simulink subsystem "VehicleSimulationRef"  (R2024a)
settings: Solver=VariableStepAuto  StartTime=0.0  StopTime=10.0  RelTol=1e-3
undefined symbols (not defined in the file): damp, Ka_accel, Kd_rate, Ki_angle, Kp_angle, omega, SimIn, SimPar
libraries: simulink_extras x3, vrlib x3, aerolibanimutils x1, simulink x1
settings Model: Creator=tbritton  LastModifiedBy=adcl
settings SolverCC: AlgebraicLoopSolver=TrustRegion
settings OptimizationCC: ReuseModelBlockBuffer=off
settings DebuggingCC: UnconnectedInputMsg=warning  UnconnectedOutputMsg=warning  UnconnectedLineMsg=warning
settings ModelReferenceCC: EnableRefExpFcnMdlSchedulingChecks=on
settings RTWCC: GPUComputeCapability=3.5  DLArmComputeVersion=19.05

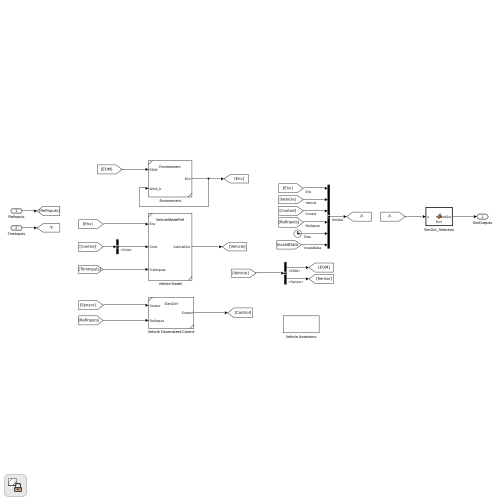
[thumbnail: Simulink's stored preview of the top-level diagram]
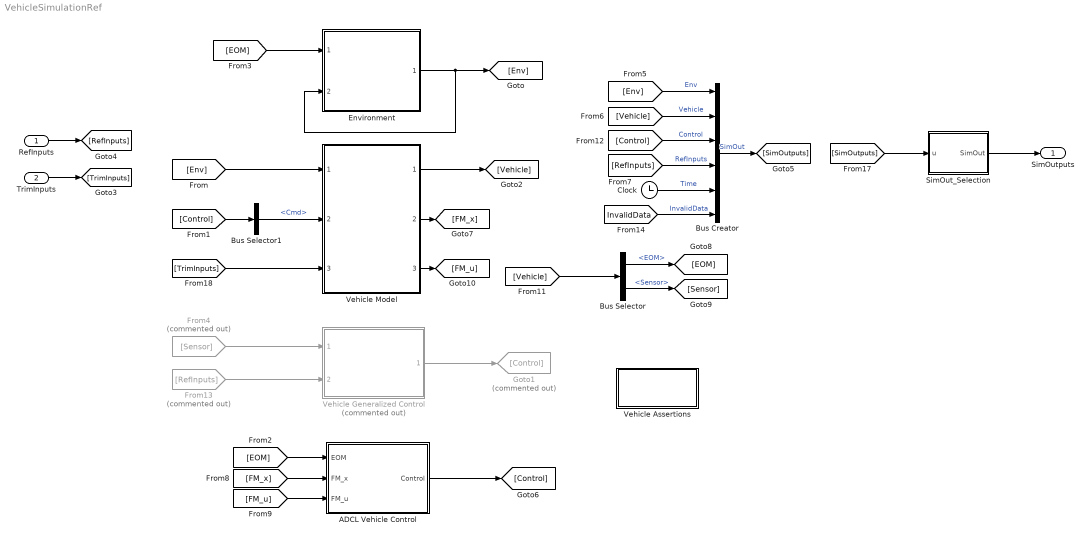
== system VehicleSimulationRef ==
  RefInputs : Inport  OutDataTypeStr=Bus: BUS_REF_INPUT
  TrimInputs : Inport  Port=2  OutDataTypeStr=Bus: BUS_TRIM_INPUT
  ADCL Vehicle Control : Subsystem
  Bus Creator : BusCreator  Inputs=6  OutDataTypeStr=Bus: BUS_SIM_OUT  NonVirtualBus=on
  Bus Selector : BusSelector  OutputSignals=EOM,Sensor
  Bus Selector1 : BusSelector  OutputSignals=Cmd
  Clock : Clock
  Environment : Subsystem  ReferencedSubsystem=Environment
  From13 : From  Commented=on  GotoTag=RefInputs
  From4 : From  Commented=on  GotoTag=Sensor
  Goto1 : Goto  Commented=on  GotoTag=Control
  SimOut_Selection : MATLAB Function  TreatAsAtomicUnit=on
  Vehicle Assertions : Subsystem
  Vehicle Generalized Control : Subsystem  Commented=on  ReferencedSubsystem=GenCtrl
  Vehicle Model : Subsystem  ReferencedSubsystem=VehicleModelRef
  SimOutputs : Outport  OutDataTypeStr=Bus: BUS_USER_SIM_OUT
  wires:
  From4/1 -> Vehicle Generalized Control/1
  [Env] -> Bus Creator/1  "Env"
  [RefInputs] -> Bus Creator/4  "RefInputs"
  Environment/1 -> [Env], Environment/2
  Vehicle Generalized Control/1 -> Goto1/1
  [Vehicle] -> Bus Creator/2  "Vehicle"
  [Control] -> Bus Creator/3  "Control"
  Bus Selector/1 -> [EOM]  "<EOM>"
  [Vehicle] -> Bus Selector/1
  [EOM] -> Environment/1
  Bus Selector/2 -> [Sensor]  "<Sensor>"
  [Control] -> Bus Selector1/1
  From13/1 -> Vehicle Generalized Control/2
  Clock/1 -> Bus Creator/5  "Time"
  TrimInputs/1 -> [TrimInputs]
  RefInputs/1 -> [RefInputs]
  Bus Creator/1 -> [SimOutputs]  "SimOut"
  [InvalidData] -> Bus Creator/6  "InvalidData"
  [Env] -> Vehicle Model/1
  Bus Selector1/1 -> Vehicle Model/2  "<Cmd>"
  [TrimInputs] -> Vehicle Model/3
  Vehicle Model/1 -> [Vehicle]
  [SimOutputs] -> SimOut_Selection/1(u)
  SimOut_Selection/1(SimOut) -> SimOutputs/1
  [EOM] -> ADCL Vehicle Control/1(EOM)
  ADCL Vehicle Control/1(Control) -> [Control]
  [FM_x] -> ADCL Vehicle Control/2(FM_x)
  [FM_u] -> ADCL Vehicle Control/3(FM_u)
  Vehicle Model/3 -> [FM_u]
  Vehicle Model/2 -> [FM_x]

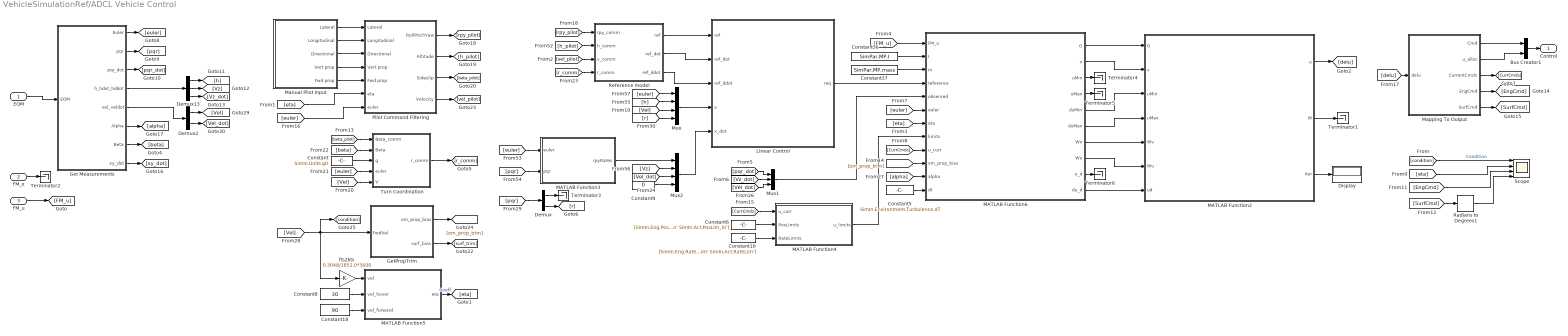
== system VehicleSimulationRef/ADCL Vehicle Control ==
  EOM : Inport
  FM_x : Inport  Port=2
  FM_u : Inport  Port=3
  Bus Creator1 : BusCreator  Inputs=2
  Constant : Constant  Value=SimIn.Units.g0
  Constant10 : Constant  Value=[SimIn.Eng.RateLim' SimIn.Act.RateLim']
  Constant18 : Constant  Value=90
  Constant36 : Constant  Value=SimPar.MP.I
  Constant37 : Constant  Value=SimPar.MP.mass
  Constant5 : Constant  Value=SimIn.Environment.Turbulence.dT
  Constant6 : Constant  Value=[SimIn.Eng.PosLim_hi' SimIn.Act.PosLim_hi'; SimIn.Eng.PosLim_lo' SimIn.Act.PosLim_lo']
  Constant8 : Constant  Value=30
  Constant9 : Constant  Value=0
  Demux : Demux  Outputs=[2 1]
  Demux13 : Demux  Outputs=3
  Demux2 : Demux  Outputs=2
  Display : Display
  Get Measurements : Subsystem
  GetPropTrim : Subsystem
  Linear Control : Subsystem  mask{Krp_angle=5, Krp_angle_i=3, Krp_rate=5, Krp_accel=1, Ky_angle=0.75, Ky_rate=2.5, Ky_accel=0.75, Kr_rate=2, Kh_angle=0.8, Kh_rate=2, Kh_accel=1}
      mask prompts: Krp_angle "Roll and Pitch angle gain"; Krp_angle_i "Roll and Pitch angle gain integral"; Krp_rate "Roll and Pitch rate gain"; Krp_accel "Roll and Pitch accel. gain"; Ky_angle "Yaw angle gain"; Ky_rate "Yaw rate gain"; Ky_accel "Yaw accel. gain"; Kr_rate "Turn coord. rate gain"; Kh_angle "Altitude angle gain"; Kh_rate "Altitude rate gain"; Kh_accel "Altitude accel. gain"
      mask DialogControl DescTextVar Prompt: Linear controller gains
      mask DialogControl Container3 Prompt: Roll and Pitch
      mask DialogControl Container4 Prompt: Yaw
      mask DialogControl Container5 Prompt: Altitude and Forward vel.
  MATLAB Function2 : MATLAB Function  TreatAsAtomicUnit=on
  MATLAB Function3 : MATLAB Function  TreatAsAtomicUnit=on
  MATLAB Function4 : MATLAB Function  TreatAsAtomicUnit=on
  MATLAB Function5 : MATLAB Function  TreatAsAtomicUnit=on
  MATLAB Function6 : MATLAB Function  TreatAsAtomicUnit=on
  Manual Pilot Input : Subsystem
  Mapping To Output : Subsystem
  Mux : Mux
  Mux1 : Mux  Inputs=3
  Mux2 : Mux
  Pilot Command Filtering : Subsystem
  Radians to Degrees1 : simulink_extras/Transformations/Radians to Degrees
  Reference model : Subsystem  mask{r_omega=1.4, r_damp=0.8, p_omega=2.4, p_damp=0.8, y_omega=0.67, y_damp=0.8, h_omega=0.67, h_damp=0.8}
      mask prompts: r_omega "Roll natural freq."; r_damp "Roll damping ratio"; p_omega "Pitch natural freq."; p_damp "Pitch damping ratio"; y_omega "Yaw natural freq."; y_damp "Yaw damping ratio"; h_omega "Altitude natural freq."; h_damp "Altitude damping ratio"
      mask DialogControl DescTextVar Prompt: Second order reference models for the roll, pitch, yaw and altitude channles
      mask DialogControl Container3 Prompt: Roll parameters
      mask DialogControl Container4 Prompt: Pitch parameters
      mask DialogControl Container5 Prompt: Yaw parameters
      mask DialogControl Container6 Prompt: Altitude parameters
  Scope : Scope  NumInputPorts=4
  Terminator{1..6} (6 alike) : Terminator
  Turn Coordination : Subsystem  mask{Kbeta=0.5}
      mask prompts: Kbeta "Controller gain"
      mask DialogControl DescTextVar Prompt: Sideslip control for turn coordination
  fts2kts : Gain  Gain=0.3048/1852.0*3600
  Control : Outport
  wires:
  MATLAB Function6/3(uMin) -> Terminator4/1
  MATLAB Function6/4(uMax) -> Terminator5/1
  MATLAB Function6/9(u_d) -> Terminator6/1
  Pilot Command Filtering/1(RollPitchYaw) -> [rpy_pilot]
  Pilot Command Filtering/2(Altitude) -> [h_pilot]
  Pilot Command Filtering/3(Sideslip) -> [beta_pilot]
  Pilot Command Filtering/4(Velocity) -> [vel_pilot]
  [euler] -> Pilot Command Filtering/7(euler)
  [eta] -> Pilot Command Filtering/6(eta)
  Manual Pilot Input/5(Fwd prop) -> Pilot Command Filtering/5(Fwd prop)
  Manual Pilot Input/4(Vert prop) -> Pilot Command Filtering/4(Vert prop)
  Manual Pilot Input/3(Directional) -> Pilot Command Filtering/3(Directional)
  Manual Pilot Input/2(Longitudinal) -> Pilot Command Filtering/2(Longitudinal)
  Manual Pilot Input/1(Lateral) -> Pilot Command Filtering/1(Lateral)
  [h] -> Mux/2
  EOM/1 -> Get Measurements/1(EOM)
  Mux/1 -> Linear Control/4(x)
  [h_pilot] -> Reference model/2(h_comm)
  Reference model/2(ref_dot) -> Linear Control/2(ref_dot)
  Reference model/3(ref_ddot) -> Linear Control/3(ref_ddot)
  [euler] -> MATLAB Function3/1(euler)
  Mux2/1 -> Linear Control/5(x_dot)
  Reference model/1(ref) -> Linear Control/1(ref)
  [pqr] -> MATLAB Function3/2(pqr)
  [euler] -> Mux/1
  [Vz] -> Mux2/2
  [rpy_pilot] -> Reference model/1(rpy_comm)
  MATLAB Function3/1(rpyRates) -> Mux2/1
  Bus Creator1/1 -> Control/1
  FM_x/1 -> Terminator2/1
  FM_u/1 -> [FM_u]
  [FM_u] -> MATLAB Function6/1(FM_u)
  Constant36/1 -> MATLAB Function6/2(I)
  Constant37/1 -> MATLAB Function6/3(m)
  [eta] -> MATLAB Function6/7(eta)
  [euler] -> MATLAB Function6/6(euler)
  MATLAB Function6/2(v) -> MATLAB Function2/2(v)
  [eta] -> Scope/2
  [SurfCmd] -> Radians to Degrees1/1
  [EngCmd] -> Scope/3
  Radians to Degrees1/1 -> Scope/4
  Get Measurements/4(h_hdot_hddot) -> Demux13/1
  Get Measurements/1(Euler) -> [euler]
  Get Measurements/2(pqr) -> [pqr]
  Get Measurements/3(pqr_dot) -> [pqr_dot]
  Demux13/1 -> [h]
  Demux13/2 -> [Vz]
  Demux13/3 -> [Vz_dot]
  Get Measurements/6(Alpha) -> [alpha]
  [om_prop_trim] -> MATLAB Function6/10(om_prop_bias)
  Mapping To Output/1(Cmd) -> Bus Creator1/1
  Mapping To Output/2(u_alloc) -> Bus Creator1/2
  Mapping To Output/3(CurrentCmds) -> [CurrCmds]
  [CurrCmds] -> MATLAB Function6/9(u_curr)
  Mapping To Output/5(SurfCmd) -> [SurfCmd]
  Mapping To Output/4(EngCmd) -> [EngCmd]
  Linear Control/1(req) -> MATLAB Function6/4(reference)
  Get Measurements/5(vel_veldot) -> Demux2/1
  Demux2/2 -> [Vel_dot]
  Demux2/1 -> [Vel]
  [Vel] -> Mux/3
  [Vel_dot] -> Mux2/3
  [alpha] -> MATLAB Function6/11(alpha)
  MATLAB Function6/1(G) -> MATLAB Function2/1(G)
  MATLAB Function6/7(Wv) -> MATLAB Function2/5(Wv)
  MATLAB Function6/8(Wu) -> MATLAB Function2/6(Wu)
  MATLAB Function6/5(duMin) -> MATLAB Function2/3(uMin)
  MATLAB Function6/6(duMax) -> MATLAB Function2/4(uMax)
  MATLAB Function5/1(eta) -> [eta]  "Coeff"
  [Vz_dot] -> Mux1/2
  [pqr_dot] -> Mux1/1
  [Vel_dot] -> Mux1/3
  Constant5/1 -> MATLAB Function6/12(dt)
  [vel_pilot] -> Reference model/3(v_comm)
  Constant6/1 -> MATLAB Function4/2(PosLimits)
  MATLAB Function4/1(u_limits) -> MATLAB Function6/8(limits)
  GetPropTrim/1(om_prop_bias) -> [om_prop_trim]
  MATLAB Function6/10(du_d) -> MATLAB Function2/7(ud)
  [Vel] -> GetPropTrim/1(FwdVel), [condition], fts2kts/1
  fts2kts/1 -> MATLAB Function5/1(vel)
  Constant8/1 -> MATLAB Function5/2(vel_hover)
  Constant18/1 -> MATLAB Function5/3(vel_forward)
  GetPropTrim/2(surf_bias) -> [surf_trim]
  [condition] -> Scope/1  "Condition"
  MATLAB Function2/3(iter) -> Display/1
  MATLAB Function2/2(W) -> Terminator1/1
  [delu] -> Mapping To Output/1(delu)
  [CurrCmds] -> MATLAB Function4/1(u_curr)
  Mux1/1 -> MATLAB Function6/5(observed)
  MATLAB Function2/1(u) -> [delu]
  Constant10/1 -> MATLAB Function4/3(RateLimits)
  [beta_pilot] -> Turn Coordination/1(Beta_comm)
  [Vel] -> Turn Coordination/5(V)
  [euler] -> Turn Coordination/4(euler)
  Get Measurements/7(Beta) -> [beta]
  [beta] -> Turn Coordination/2(Beta)
  Constant/1 -> Turn Coordination/3(g)
  [r_comm] -> Reference model/4(r_comm)
  [pqr] -> Demux/1
  Demux/2 -> [r]
  Demux/1 -> Terminator3/1
  [r] -> Mux/4
  Constant9/1 -> Mux2/4
  Turn Coordination/1(r_comm) -> [r_comm]
  Get Measurements/8(xy_dot) -> [xy_dot]

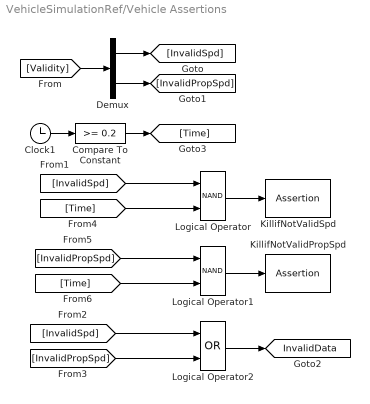
== system VehicleSimulationRef/Vehicle Assertions ==
  Clock1 : Clock
  Compare To Constant : simulink/Logic and Bit Operations/Compare To Constant  relop=>=  const=0.2  OutDataTypeStr=boolean  ZeroCross=off
  Demux : Demux  Outputs=2
  KillifNotValidPropSpd : Assertion  AssertionFailFcn=warndlg('Model invalid prop speeds','Warning!')
  KillifNotValidSpd : Assertion  AssertionFailFcn=warndlg('Model invalid speed','Warning!')
  Logical Operator : Logic  Operator=NAND  AllPortsSameDT=off  OutDataTypeStr=boolean
  Logical Operator1 : Logic  Operator=NAND  AllPortsSameDT=off  OutDataTypeStr=boolean
  Logical Operator2 : Logic  Operator=OR  AllPortsSameDT=off  OutDataTypeStr=boolean
  tag scope: InvalidData=global
  wires:
  [InvalidPropSpd] -> Logical Operator2/2
  [InvalidSpd] -> Logical Operator2/1
  Logical Operator2/1 -> [InvalidData]
  Logical Operator/1 -> KillifNotValidSpd/1
  [InvalidPropSpd] -> Logical Operator1/1
  Logical Operator1/1 -> KillifNotValidPropSpd/1
  [Time] -> Logical Operator1/2
  [Time] -> Logical Operator/2
  Compare To Constant/1 -> [Time]
  Demux/2 -> [InvalidPropSpd]
  Demux/1 -> [InvalidSpd]
  [Validity] -> Demux/1
  [InvalidSpd] -> Logical Operator/1
  Clock1/1 -> Compare To Constant/1

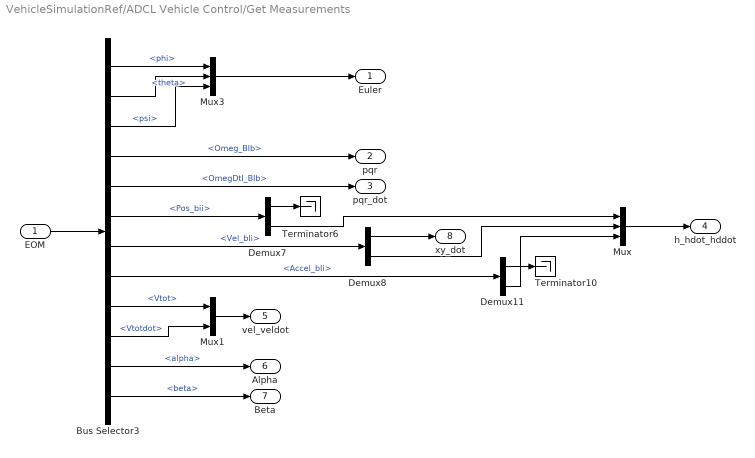
== system VehicleSimulationRef/ADCL Vehicle Control/Get Measurements ==
  EOM : Inport
  Bus Selector3 : BusSelector  OutputSignals=WorldRelativeData.Euler.phi,WorldRelativeData.Euler.theta,WorldRelativeData.Euler.psi,InertialData.Omeg_BIb,InertialData.OmegDtI_BIb,InertialData.Pos_bii,InertialData.Vel_bIi,InertialData.Accel_bIi,AirRelativeData.Vtot,AirRelativeData.Vtotdot,AirRelativeData.alpha,AirRelativeData.beta
  Demux11 : Demux  Outputs=[2 1]
  Demux7 : Demux  Outputs=[2 1]
  Demux8 : Demux  Outputs=[2 1]
  Mux : Mux  Inputs=3
  Mux1 : Mux  Inputs=2
  Mux3 : Mux  Inputs=3
  Terminator10 : Terminator
  Terminator6 : Terminator
  Euler : Outport
  pqr : Outport  Port=2
  pqr_dot : Outport  Port=3
  h_hdot_hddot : Outport  Port=4
  vel_veldot : Outport  Port=5
  Alpha : Outport  Port=6
  Beta : Outport  Port=7
  xy_dot : Outport  Port=8
  wires:
  Bus Selector3/7 -> Demux8/1  "<Vel_bIi>"
  Bus Selector3/6 -> Demux7/1  "<Pos_bii>"
  EOM/1 -> Bus Selector3/1
  Demux7/1 -> Terminator6/1
  Bus Selector3/8 -> Demux11/1  "<Accel_bIi>"
  Bus Selector3/1 -> Mux3/1  "<phi>"
  Demux11/1 -> Terminator10/1
  Demux11/2 -> Mux/3
  Demux7/2 -> Mux/1
  Bus Selector3/2 -> Mux3/2  "<theta>"
  Bus Selector3/3 -> Mux3/3  "<psi>"
  Mux3/1 -> Euler/1
  Bus Selector3/4 -> pqr/1  "<Omeg_BIb>"
  Bus Selector3/5 -> pqr_dot/1  "<OmegDtI_BIb>"
  Mux/1 -> h_hdot_hddot/1
  Demux8/2 -> Mux/2
  Bus Selector3/11 -> Alpha/1  "<alpha>"
  Bus Selector3/10 -> Mux1/2  "<Vtotdot>"
  Bus Selector3/9 -> Mux1/1  "<Vtot>"
  Mux1/1 -> vel_veldot/1
  Bus Selector3/12 -> Beta/1  "<beta>"
  Demux8/1 -> xy_dot/1

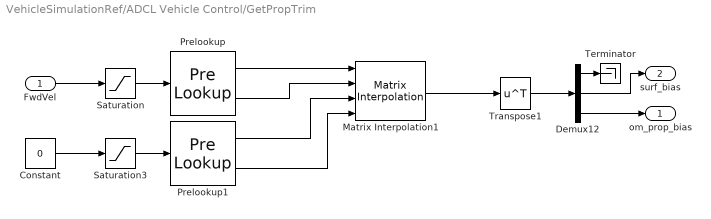
== system VehicleSimulationRef/ADCL Vehicle Control/GetPropTrim ==
  FwdVel : Inport
  Constant : Constant  Value=0
  Demux12 : Demux  Outputs=[12 4 9]
  Matrix Interpolation1 : simulink_extras/Additional Lookup Tables/Matrix Interpolation  InterpMethod=Linear  ExtrapMethod=Clip  InterpolateDimension=2  TableData=SimIn.Control.trim.XU0_interp  SimulateUsing=Code generation
  Prelookup : PreLookup  BreakpointsData=SimIn.Control.trim.UH
  Prelookup1 : PreLookup  BreakpointsData=SimIn.Control.trim.WH
  Saturation : Saturate  UpperLimit=178  LowerLimit=0
  Saturation3 : Saturate  UpperLimit=8.33  LowerLimit=-8.33
  Terminator : Terminator
  Transpose1 : Math  Operator=transpose
  om_prop_bias : Outport
  surf_bias : Outport  Port=2
  wires:
  Constant/1 -> Saturation3/1
  Prelookup/1 -> Matrix Interpolation1/1
  Prelookup1/1 -> Matrix Interpolation1/3
  Demux12/2 -> surf_bias/1
  Demux12/3 -> om_prop_bias/1
  Demux12/1 -> Terminator/1
  Prelookup/2 -> Matrix Interpolation1/2
  Prelookup1/2 -> Matrix Interpolation1/4
  Transpose1/1 -> Demux12/1
  Saturation/1 -> Prelookup/1
  Saturation3/1 -> Prelookup1/1
  FwdVel/1 -> Saturation/1
  Matrix Interpolation1/1 -> Transpose1/1

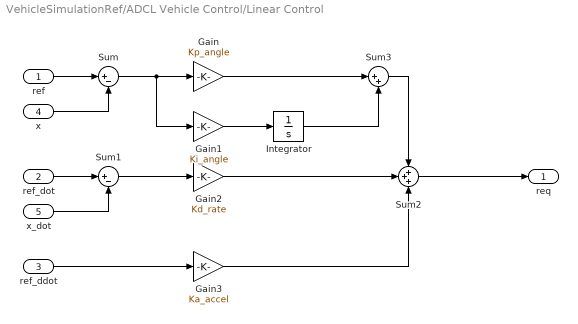
== system VehicleSimulationRef/ADCL Vehicle Control/Linear Control ==
  ref : Inport
  ref_dot : Inport  Port=2
  ref_ddot : Inport  Port=3
  x : Inport  Port=4
  x_dot : Inport  Port=5
  Gain : Gain  Gain=Kp_angle
  Gain1 : Gain  Gain=Ki_angle
  Gain2 : Gain  Gain=Kd_rate
  Gain3 : Gain  Gain=Ka_accel
  Integrator : Integrator
  Sum : Sum  Inputs=|+-
  Sum1 : Sum  Inputs=|+-
  Sum2 : Sum  Inputs=+++
  Sum3 : Sum  Inputs=|++
  req : Outport
  wires:
  ref/1 -> Sum/1
  x/1 -> Sum/2
  Gain1/1 -> Integrator/1
  Sum/1 -> Gain/1, Gain1/1
  ref_dot/1 -> Sum1/1
  Sum1/1 -> Gain2/1
  x_dot/1 -> Sum1/2
  ref_ddot/1 -> Gain3/1
  Gain3/1 -> Sum2/3
  Gain2/1 -> Sum2/2
  Gain/1 -> Sum3/1
  Integrator/1 -> Sum3/2
  Sum3/1 -> Sum2/1
  Sum2/1 -> req/1

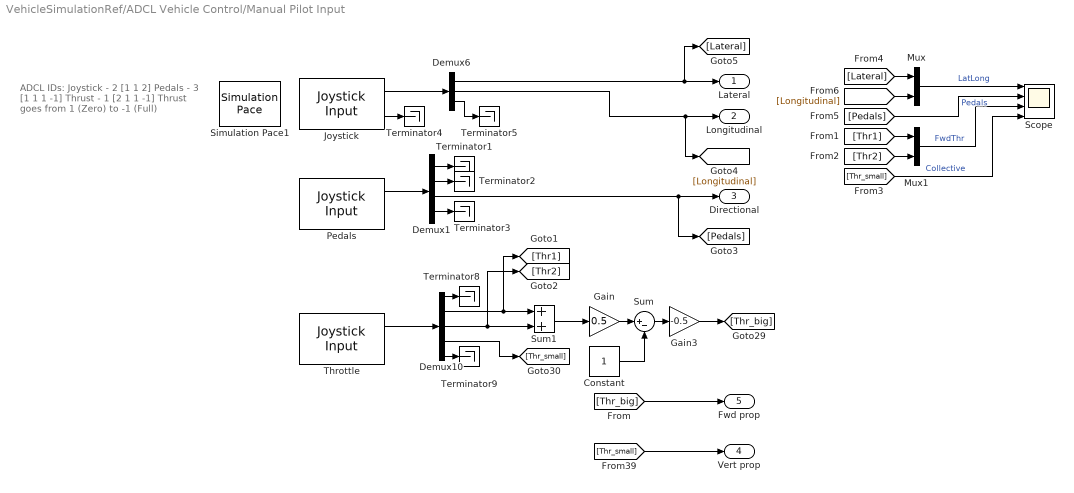
== system VehicleSimulationRef/ADCL Vehicle Control/Manual Pilot Input ==
  note: ADCL IDs:
      | Joystick - 2 [1 1 2]
      | Pedals - 3 [1 1 1 -1]
      | Thrust - 1 [2 1 1 -1]
      |
      | Thrust goes from 1 (Zero) to -1 (Full)
  Constant : Constant
  Demux1 : Demux  Outputs=[1 1 1 -1]
  Demux10 : Demux  Outputs=[2 1 1 1 2]
  Demux6 : Demux  Outputs=[1 1 2]
  Gain : Gain  Gain=0.5
  Gain3 : Gain  Gain=-0.5
  Joystick : vrlib/Joystick Input  joyid=2  adjustports=on  forcefeed=off
  Mux : Mux  Inputs=2
  Mux1 : Mux  Inputs=2
  Pedals : vrlib/Joystick Input  joyid=3  adjustports=off  forcefeed=off
  Scope : Scope  NumInputPorts=4
  Simulation Pace1 : aerolibanimutils/Simulation Pace  SimulationPace=1  SleepMode=Auto  OutputPaceError=off  SampleTime=SimIn.Environment.Turbulence.dT
  Sum : Sum  Inputs=|+-
  Sum1 : Sum
  Terminator{1..5,8..9} (7 alike) : Terminator
  Throttle : vrlib/Joystick Input  joyid=1  adjustports=on  forcefeed=off
  Lateral : Outport
  Longitudinal : Outport  Port=2
  Directional : Outport  Port=3
  Vert prop : Outport  Port=4
  Fwd prop : Outport  Port=5
  wires:
  [Thr_small] -> Scope/4  "Collective"
  Mux1/1 -> Scope/3  "FwdThr"
  [Pedals] -> Scope/2  "Pedals"
  Mux/1 -> Scope/1  "LatLong"
  [Thr2] -> Mux1/2
  [Thr1] -> Mux1/1
  [Lateral] -> Mux/1
  [Longitudinal] -> Mux/2
  Demux1/3 -> Directional/1, [Pedals]
  [Thr_small] -> Vert prop/1
  [Thr_big] -> Fwd prop/1
  Demux6/2 -> Longitudinal/1, [Longitudinal]
  Demux1/1 -> Terminator1/1
  Demux1/2 -> Terminator2/1
  Demux1/4 -> Terminator3/1
  Pedals/1 -> Demux1/1
  Gain3/1 -> [Thr_big]
  Constant/1 -> Sum/2
  Sum/1 -> Gain3/1
  Demux6/3 -> Terminator5/1
  Demux6/1 -> Lateral/1, [Lateral]
  Joystick/1 -> Demux6/1
  Throttle/1 -> Demux10/1
  Sum1/1 -> Gain/1
  Demux10/2 -> Sum1/1, [Thr1]
  Demux10/5 -> Terminator9/1
  Gain/1 -> Sum/1
  Demux10/1 -> Terminator8/1
  Demux10/3 -> Sum1/2, [Thr2]
  Demux10/4 -> [Thr_small]
  Joystick/2 -> Terminator4/1

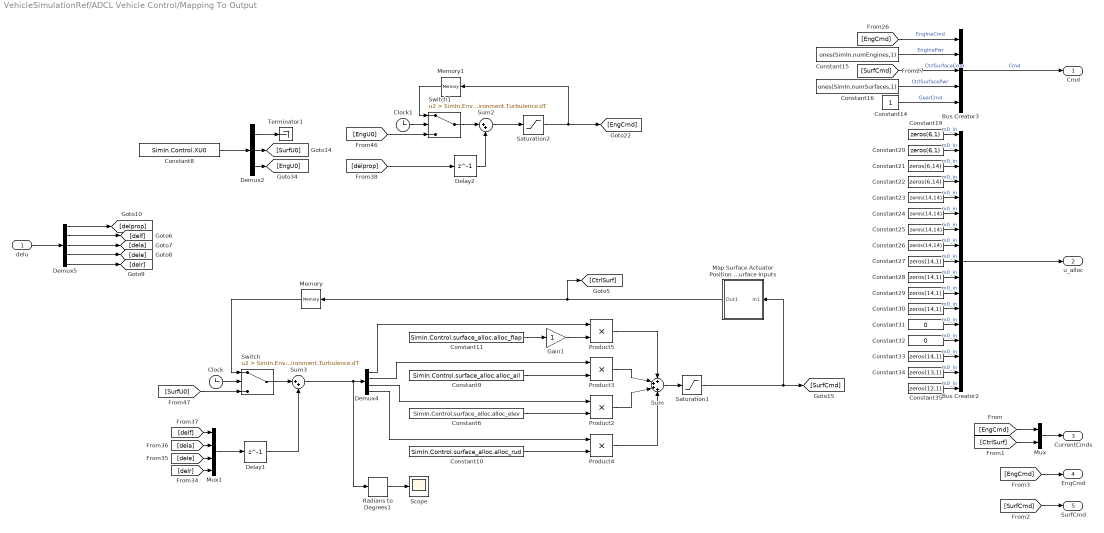
== system VehicleSimulationRef/ADCL Vehicle Control/Mapping To Output ==
  delu : Inport
  Bus Creator2 : BusCreator  Inputs=17  OutDataTypeStr=Bus: BUS_ALLOC
  Bus Creator3 : BusCreator  Inputs=5  OutDataTypeStr=Bus: BUS_CMD
  Clock : Clock
  Clock1 : Clock
  Constant10 : Constant  Value=SimIn.Control.surface_alloc.alloc_rud
  Constant11 : Constant  Value=SimIn.Control.surface_alloc.alloc_flap
  Constant14 : Constant
  Constant15 : Constant  Value=ones(SimIn.numEngines,1)
  Constant16 : Constant  Value=ones(SimIn.numSurfaces,1)
  Constant19 : Constant  Value=zeros(6,1)
  Constant20 : Constant  Value=zeros(6,1)
  Constant21 : Constant  Value=zeros(6,14)
  Constant22 : Constant  Value=zeros(6,14)
  Constant{23..26} (4 alike) : Constant  Value=zeros(14,14)
  Constant{27..30,33} (5 alike) : Constant  Value=zeros(14,1)
  Constant31 : Constant  Value=0
  Constant32 : Constant  Value=0
  Constant34 : Constant  Value=zeros(13,1)
  Constant35 : Constant  Value=zeros(12,1)
  Constant6 : Constant  Value=SimIn.Control.surface_alloc.alloc_elev
  Constant8 : Constant  Value=SimIn.Control.XU0
  Constant9 : Constant  Value=SimIn.Control.surface_alloc.alloc_ail
  Delay1 : Delay  DelayLength=1
  Delay2 : Delay  DelayLength=1
  Demux2 : Demux  Outputs=[-1 4 9]
  Demux4 : Demux
  Demux5 : Demux  Outputs=[9 1 1 1 1]
  Gain1 : Gain
  Map Surface Actuator Position To Surface Inputs : Subsystem
  Memory : Memory
  Memory1 : Memory
  Mux : Mux  Inputs=2
  Mux1 : Mux
  Product{2..5} (4 alike) : Product
  Radians to Degrees1 : simulink_extras/Transformations/Radians to Degrees
  Saturation1 : Saturate  UpperLimit=SimPar.Actuator.MaxPos  LowerLimit=SimPar.Actuator.MinPos
  Saturation2 : Saturate  UpperLimit=SimPar.Engine.MaxPos  LowerLimit=SimPar.Engine.MinPos
  Scope : Scope
  Sum : Sum  Inputs=++++
  Sum2 : Sum  Inputs=|++
  Sum3 : Sum  Inputs=|++
  Switch : Switch  Criteria=u2 > Threshold  Threshold=SimIn.Environment.Turbulence.dT  SaturateOnIntegerOverflow=off  InputSameDT=off
  Switch1 : Switch  Criteria=u2 > Threshold  Threshold=SimIn.Environment.Turbulence.dT  SaturateOnIntegerOverflow=off  InputSameDT=off
  Terminator1 : Terminator
  Cmd : Outport
  u_alloc : Outport  Port=2
  CurrentCmds : Outport  Port=3
  EngCmd : Outport  Port=4
  SurfCmd : Outport  Port=5
  wires:
  Constant6/1 -> Product2/2
  Switch/1 -> Sum3/1
  Bus Creator3/1 -> Cmd/1  "Cmd"
  Demux4/2 -> Product3/1
  Constant31/1 -> Bus Creator2/13  "m0_in"
  [SurfCmd] -> Bus Creator3/3  "CtrlSurfaceCmd"
  [SurfU0] -> Switch/3
  Constant26/1 -> Bus Creator2/8  "m0_in"
  Demux4/4 -> Product4/1
  Delay1/1 -> Sum3/2
  Constant9/1 -> Product3/2
  [EngCmd] -> Bus Creator3/1  "EngineCmd"
  Product5/1 -> Sum/1
  [delf] -> Mux1/1
  Constant24/1 -> Bus Creator2/6  "m0_in"
  [dela] -> Mux1/2
  Mux1/1 -> Delay1/1
  Product2/1 -> Sum/3
  Memory1/1 -> Switch1/1
  Demux2/1 -> Terminator1/1
  [delr] -> Mux1/4
  Sum/1 -> Saturation1/1
  Constant19/1 -> Bus Creator2/1  "m0_in"
  Constant22/1 -> Bus Creator2/4  "m0_in"
  Constant33/1 -> Bus Creator2/15  "m0_in"
  Switch1/1 -> Sum2/1
  Product4/1 -> Sum/4
  Constant20/1 -> Bus Creator2/2  "m0_in"
  Constant28/1 -> Bus Creator2/10  "m0_in"
  Gain1/1 -> Product5/2
  Clock1/1 -> Switch1/2
  Demux2/2 -> [SurfU0]
  Demux4/3 -> Product2/1
  Clock/1 -> Switch/2
  Constant16/1 -> Bus Creator3/4  "CtrlSurfacePwr"
  Demux2/3 -> [EngU0]
  Constant27/1 -> Bus Creator2/9  "m0_in"
  Constant11/1 -> Gain1/1
  Saturation1/1 -> Map Surface Actuator Position To Surface Inputs/1(In1), [SurfCmd]
  [EngU0] -> Switch1/3
  Constant29/1 -> Bus Creator2/11  "m0_in"
  Constant8/1 -> Demux2/1
  [dele] -> Mux1/3
  Product3/1 -> Sum/2
  Constant32/1 -> Bus Creator2/14  "m0_in"
  Bus Creator2/1 -> u_alloc/1
  Constant15/1 -> Bus Creator3/2  "EnginePwr"
  Constant30/1 -> Bus Creator2/12  "m0_in"
  Memory/1 -> Switch/1
  Sum3/1 -> Radians to Degrees1/1, Demux4/1
  Constant25/1 -> Bus Creator2/7  "m0_in"
  Saturation2/1 -> Memory1/1, [EngCmd]
  Demux4/1 -> Product5/1
  Constant35/1 -> Bus Creator2/17  "m0_in"
  Delay2/1 -> Sum2/2
  Constant14/1 -> Bus Creator3/5  "GearCmd"
  Constant23/1 -> Bus Creator2/5  "m0_in"
  Constant21/1 -> Bus Creator2/3  "m0_in"
  Constant10/1 -> Product4/2
  Constant34/1 -> Bus Creator2/16  "m0_in"
  [delprop] -> Delay2/1
  Sum2/1 -> Saturation2/1
  Mux/1 -> CurrentCmds/1
  [EngCmd] -> Mux/1
  [CtrlSurf] -> Mux/2
  [SurfCmd] -> SurfCmd/1
  [EngCmd] -> EngCmd/1
  Map Surface Actuator Position To Surface Inputs/1(Out1) -> [CtrlSurf], Memory/1
  Demux5/2 -> [delf]
  delu/1 -> Demux5/1
  Demux5/1 -> [delprop]
  Demux5/3 -> [dela]
  Demux5/4 -> [dele]
  Demux5/5 -> [delr]
  Radians to Degrees1/1 -> Scope/1

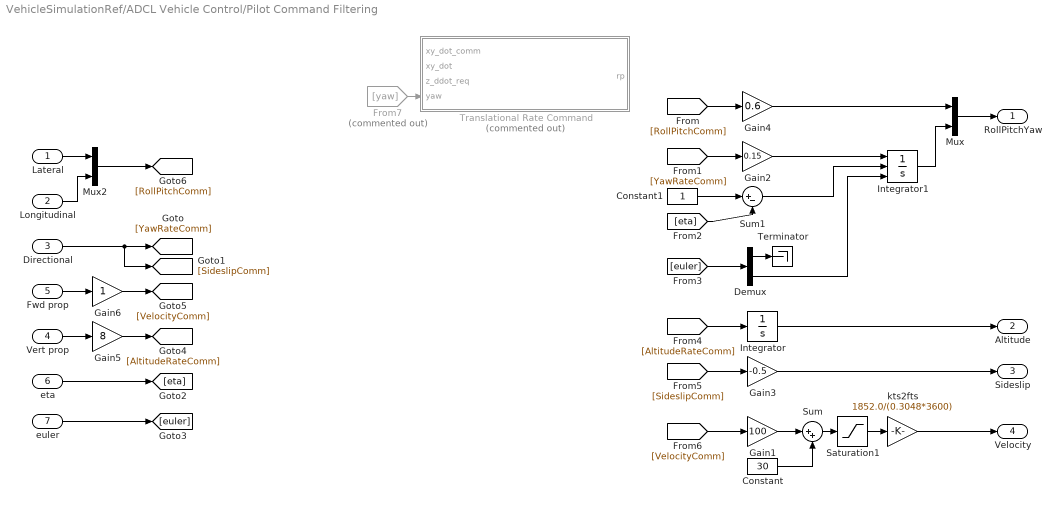
== system VehicleSimulationRef/ADCL Vehicle Control/Pilot Command Filtering ==
  Lateral : Inport
  Longitudinal : Inport  Port=2
  Directional : Inport  Port=3
  Vert prop : Inport  Port=4
  Fwd prop : Inport  Port=5
  eta : Inport  Port=6
  euler : Inport  Port=7
  Constant : Constant  Value=30
  Constant1 : Constant
  Demux : Demux  Outputs=[2 1]
  From7 : From  Commented=on  GotoTag=yaw
  Gain1 : Gain  Gain=100
  Gain2 : Gain  Gain=0.15
  Gain3 : Gain  Gain=-0.5
  Gain4 : Gain  Gain=0.6
  Gain5 : Gain  Gain=8
  Gain6 : Gain
  Integrator : Integrator
  Integrator1 : Integrator  ExternalReset=level  InitialConditionSource=external  LimitOutput=on  UpperSaturationLimit=deg2rad(175)  LowerSaturationLimit=-deg2rad(175)
  Mux : Mux  Inputs=2
  Mux2 : Mux  Inputs=2
  Saturation1 : Saturate  UpperLimit=130  LowerLimit=30
  Sum : Sum  Inputs=|++
  Sum1 : Sum  Inputs=|+-
  Terminator : Terminator
  Translational Rate Command : Subsystem  Commented=on
  kts2fts : Gain  Gain=1852.0/(0.3048*3600)
  RollPitchYaw : Outport
  Altitude : Outport  Port=2
  Sideslip : Outport  Port=3
  Velocity : Outport  Port=4
  wires:
  Gain4/1 -> Mux/1
  Sum1/1 -> Integrator1/2
  [eta] -> Sum1/2
  Constant1/1 -> Sum1/1
  Gain3/1 -> Sideslip/1
  Demux/1 -> Terminator/1
  Demux/2 -> Integrator1/3
  [euler] -> Demux/1
  [SideslipComm] -> Gain3/1
  Gain2/1 -> Integrator1/1
  kts2fts/1 -> Velocity/1
  Sum/1 -> Saturation1/1
  Gain1/1 -> Sum/1
  [VelocityComm] -> Gain1/1
  Constant/1 -> Sum/2
  Saturation1/1 -> kts2fts/1
  Integrator1/1 -> Mux/2
  Integrator/1 -> Altitude/1
  [AltitudeRateComm] -> Integrator/1
  Mux/1 -> RollPitchYaw/1
  [RollPitchComm] -> Gain4/1
  [YawRateComm] -> Gain2/1
  Directional/1 -> [YawRateComm], [SideslipComm]
  euler/1 -> [euler]
  eta/1 -> [eta]
  Vert prop/1 -> Gain5/1
  Gain5/1 -> [AltitudeRateComm]
  Fwd prop/1 -> Gain6/1
  Lateral/1 -> Mux2/1
  Longitudinal/1 -> Mux2/2
  Mux2/1 -> [RollPitchComm]
  Gain6/1 -> [VelocityComm]
  From7/1 -> Translational Rate Command/4(yaw)

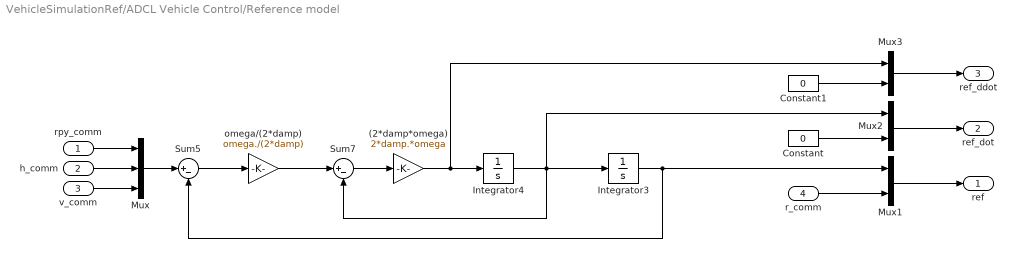
== system VehicleSimulationRef/ADCL Vehicle Control/Reference model ==
  rpy_comm : Inport
  h_comm : Inport  Port=2
  v_comm : Inport  Port=3
  r_comm : Inport  Port=4
  (2*damp*omega) : Gain  Gain=2*damp.*omega
  Constant : Constant  Value=0
  Constant1 : Constant  Value=0
  Integrator3 : Integrator
  Integrator4 : Integrator
  Mux : Mux  Inputs=3
  Mux1 : Mux  Inputs=2
  Mux2 : Mux  Inputs=2
  Mux3 : Mux  Inputs=2
  Sum5 : Sum  Inputs=|+-
  Sum7 : Sum  Inputs=|+-
  omega/(2*damp) : Gain  Gain=omega./(2*damp)
  ref : Outport
  ref_dot : Outport  Port=2
  ref_ddot : Outport  Port=3
  wires:
  rpy_comm/1 -> Mux/1
  h_comm/1 -> Mux/2
  Sum5/1 -> omega/(2*damp)/1
  Sum7/1 -> (2*damp*omega)/1
  omega/(2*damp)/1 -> Sum7/1
  (2*damp*omega)/1 -> Mux3/1, Integrator4/1
  Mux/1 -> Sum5/1
  Integrator3/1 -> Sum5/2, Mux1/1
  Integrator4/1 -> Mux2/1, Integrator3/1, Sum7/2
  v_comm/1 -> Mux/3
  r_comm/1 -> Mux1/2
  Mux1/1 -> ref/1
  Mux2/1 -> ref_dot/1
  Mux3/1 -> ref_ddot/1
  Constant1/1 -> Mux3/2
  Constant/1 -> Mux2/2

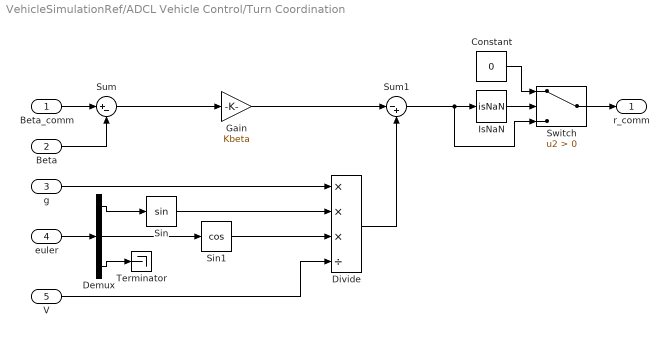
== system VehicleSimulationRef/ADCL Vehicle Control/Turn Coordination ==
  Beta_comm : Inport
  Beta : Inport  Port=2
  g : Inport  Port=3
  euler : Inport  Port=4
  V : Inport  Port=5
  Constant : Constant  Value=0
  Demux : Demux  Outputs=3
  Divide : Product  Inputs=***/
  Gain : Gain  Gain=Kbeta
  IsNaN : RelationalOperator  Operator=isNaN  OutDataTypeStr=boolean  RndMeth=Simplest  InputSameDT=off
  Sin : Trigonometry
  Sin1 : Trigonometry  Operator=cos
  Sum : Sum  Inputs=|+-
  Sum1 : Sum  Inputs=|-+
  Switch : Switch  Criteria=u2 > Threshold  SaturateOnIntegerOverflow=off  InputSameDT=off
  Terminator : Terminator
  r_comm : Outport
  wires:
  Beta_comm/1 -> Sum/1
  Beta/1 -> Sum/2
  Sum/1 -> Gain/1
  euler/1 -> Demux/1
  Demux/1 -> Sin/1
  Demux/2 -> Sin1/1
  g/1 -> Divide/1
  Sin/1 -> Divide/2
  Sin1/1 -> Divide/3
  V/1 -> Divide/4
  Divide/1 -> Sum1/2
  Demux/3 -> Terminator/1
  Gain/1 -> Sum1/1
  Switch/1 -> r_comm/1
  IsNaN/1 -> Switch/2
  Sum1/1 -> Switch/3, IsNaN/1
  Constant/1 -> Switch/1

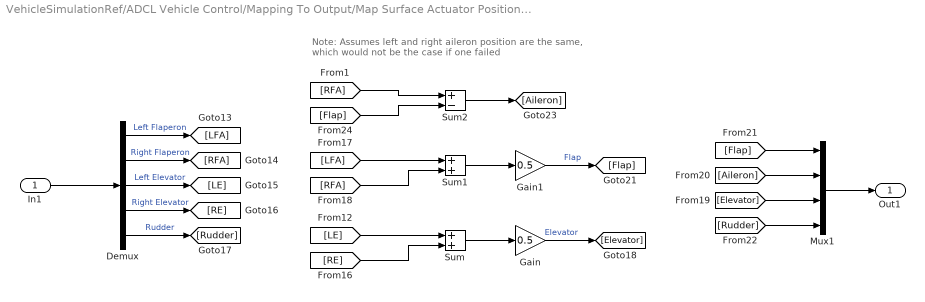
== system VehicleSimulationRef/ADCL Vehicle Control/Mapping To Output/Map Surface Actuator Position To Surface Inputs ==
  note: Note:  Assumes left and right aileron position are the same,
      |           which would not be the case if one failed
  In1 : Inport
  Demux : Demux  Outputs=SimIn.numSurfaces
  Gain : Gain  Gain=0.5
  Gain1 : Gain  Gain=0.5
  Mux1 : Mux
  Sum : Sum
  Sum1 : Sum
  Sum2 : Sum  Inputs=+-
  Out1 : Outport
  wires:
  In1/1 -> Demux/1
  [Flap] -> Sum2/2
  Sum/1 -> Gain/1
  [RE] -> Sum/2
  Demux/3 -> [LE]  "Left Elevator"
  [LFA] -> Sum1/1
  Sum1/1 -> Gain1/1
  Sum2/1 -> [Aileron]
  Demux/4 -> [RE]  "Right Elevator"
  Gain/1 -> [Elevator]  "Elevator"
  [Rudder] -> Mux1/4
  Demux/5 -> [Rudder]  "Rudder"
  Demux/2 -> [RFA]  "Right Flaperon"
  [RFA] -> Sum1/2
  Mux1/1 -> Out1/1
  Demux/1 -> [LFA]  "Left Flaperon"
  [RFA] -> Sum2/1
  [LE] -> Sum/1
  [Elevator] -> Mux1/3
  Gain1/1 -> [Flap]  "Flap"
  [Aileron] -> Mux1/2
  [Flap] -> Mux1/1

== system VehicleSimulationRef/ADCL Vehicle Control/Pilot Command Filtering/Translational Rate Command ==
  xy_dot_comm : Inport
  xy_dot : Inport  Port=2
  z_ddot_req : Inport  Port=3
  yaw : Inport  Port=4
  Constant : Constant  Value=SimIn.Units.g0
  Linear controller : Subsystem  mask{Kp=[0.5; 0.5], Ki=[0.25^2; 0.25^2], Ka=[1; 1]}
      mask prompts: Kp "Rate gain"; Ki "Rate integral gain"; Ka "Acceleration gain"
      mask DialogControl DescTextVar Prompt: Linear controllers of the two TRC channels
  MATLAB Function : MATLAB Function  TreatAsAtomicUnit=on
  Reference model : Subsystem  mask{Tv=3}
      mask prompts: Tv "Time constant"
      mask DialogControl DescTextVar Prompt: First order reference models for the two TRC channels
  rp : Outport
  wires:
  Constant/1 -> MATLAB Function/4(g)
  yaw/1 -> MATLAB Function/3(yaw)
  z_ddot_req/1 -> MATLAB Function/2(z_req)
  Linear controller/1(req) -> MATLAB Function/1(xy_req)
  MATLAB Function/1(rp) -> rp/1
  xy_dot/1 -> Linear controller/3(x_dot)
  Reference model/2(ref_dot) -> Linear controller/2(ref_dot)
  Reference model/1(ref) -> Linear controller/1(ref)
  xy_dot_comm/1 -> Reference model/1(xy_dot_comm)

== system VehicleSimulationRef/ADCL Vehicle Control/Pilot Command Filtering/Translational Rate Command/Linear controller ==
  ref : Inport
  ref_dot : Inport  Port=2
  x_dot : Inport  Port=3
  Gain : Gain  Gain=Kp
  Gain1 : Gain  Gain=Ki
  Gain2 : Gain  Gain=Ka
  Integrator : Integrator
  Sum : Sum  Inputs=|+-
  Sum1 : Sum  Inputs=+++
  req : Outport
  wires:
  Gain2/1 -> Sum1/1
  ref_dot/1 -> Gain2/1
  Integrator/1 -> Sum1/3
  Gain/1 -> Sum1/2
  Sum1/1 -> req/1
  Gain1/1 -> Integrator/1
  Sum/1 -> Gain/1, Gain1/1
  x_dot/1 -> Sum/2
  ref/1 -> Sum/1

== system VehicleSimulationRef/ADCL Vehicle Control/Pilot Command Filtering/Translational Rate Command/Reference model ==
  xy_dot_comm : Inport
  1/Tv : Gain  Gain=1/Tv
  Integrator : Integrator
  Sum : Sum  Inputs=|+-
  ref : Outport
  ref_dot : Outport  Port=2
  wires:
  Sum/1 -> 1/Tv/1
  xy_dot_comm/1 -> Sum/1
  1/Tv/1 -> Integrator/1, ref_dot/1
  Integrator/1 -> ref/1, Sum/2

== matlab function VehicleSimulationRef/ADCL Vehicle Control/MATLAB Function4 ==
  data: u_curr input; u_limits output; PosLimits input; RateLimits input
function u_limits   = limitFlaperon(u_curr, PosLimits, RateLimits)
    u_limits   = limitFlap(u_curr, PosLimits, RateLimits);
end

== matlab function VehicleSimulationRef/SimOut_Selection ==
  data: u input; SimOut output Bus: BUS_USER_SIM_OUT
function SimOut = fcn(u)

SimOut = mySimOutFunc(u);

== matlab function VehicleSimulationRef/ADCL Vehicle Control/Pilot Command Filtering/Translational Rate Command/MATLAB Function ==
  data: xy_req input; rp output; z_req input; yaw input; g input
function rp = inversion(xy_req, z_req, yaw, g)
    % Extract x and y accelerations
    ddot_x = xy_req(1);
    ddot_y = xy_req(2);

    % z acceleration
    ddot_z = z_req;

    % Compute theta_req
    theta_req = atan2( (ddot_x*cos(yaw) + ddot_y*sin(yaw)), (ddot_z - g) );

    % Compute phi_req
    phi_req = -asin( (ddot_y*cos(yaw) - ddot_x*sin(yaw)) / ...
                     sqrt(ddot_x^2 + ddot_y^2 + (ddot_z - g)^2) );

    rp = [phi_req; theta_req];
end

== matlab function VehicleSimulationRef/ADCL Vehicle Control/MATLAB Function2 ==
  data: G input; v input; uMin input; u output; uMax input; Wv input; Wu input; ud input; W output; iter output
function [u, W, iter] = runWLS(G, v, uMin, uMax, Wv, Wu, ud)
    [u, W, iter] = activeSetWLS(G, v, uMin, uMax, Wv, Wu, ud);
end

== matlab function VehicleSimulationRef/ADCL Vehicle Control/MATLAB Function3 ==
  data: euler input; rpyRates output; pqr input
function rpyRates = rpyRates(euler, pqr)
    rpyRates = euler_rates(euler, pqr);
end

== matlab function VehicleSimulationRef/ADCL Vehicle Control/MATLAB Function5 ==
  data: eta output; vel input; vel_hover input; vel_forward input
function eta = getBlendingCoeff(vel,  vel_hover, vel_forward)
    eta = blendingCoeff(vel,  vel_hover, vel_forward);
end

== matlab function VehicleSimulationRef/ADCL Vehicle Control/MATLAB Function6 ==
  data: G output; v output; FM_u input; uMin output; I input; m input; reference input; observed input; euler input; eta input; limits input; u_curr input; om_prop_bias input; alpha input; dt input; uMax output; duMin output; duMax output; Wv output; Wu output; u_d output; du_d output
function [G, v, uMin, uMax, duMin, duMax, Wv, Wu, u_d, du_d] = setupWLS(FM_u, I, m, reference, observed, euler, eta, limits, u_curr, om_prop_bias, alpha, dt)
    [G, v, uMin, uMax, duMin, duMax, Wv, Wu, u_d, du_d] = INDI_control(FM_u, I, m, reference, observed, euler, eta, limits, u_curr, om_prop_bias, alpha, dt);
end
